simulink model "DC_Motor_BrakeMode"  (R2019b)
settings: Solver=VariableStepAuto  StartTime=0.0  StopTime=10.0  FixedStep=1e-5  RelTol=1e-3
PreLoadFcn:
  | modelDir = fileparts(get_param(bdroot, 'FileName'));
  | addpath(fullfile(modelDir,'../../Parameters'));
  | 
  | Parameters_Model
  | Parameters_Simulation
  | Parameters_Controller
InitFcn:
  | Parameters_Model
  | Parameters_Simulation
  | Parameters_Controller
undefined symbols (not defined in the file): B, dTheta0, I0, J, Ke, Kt, L, R, tau_c, theta0
settings Model: Creator=Thomas  LastModifiedBy=thomas.jespersen
settings DataIOCC: ReturnWorkspaceOutputs=off
settings DebuggingCC: ArithmeticOperatorsInVariantConditions=warning
settings SFSimCC: SimUseLocalCustomCode=off  CustomCodeUndefinedFunction=UseInterfaceOnly
settings RTWCC: RTWUseLocalCustomCode=off

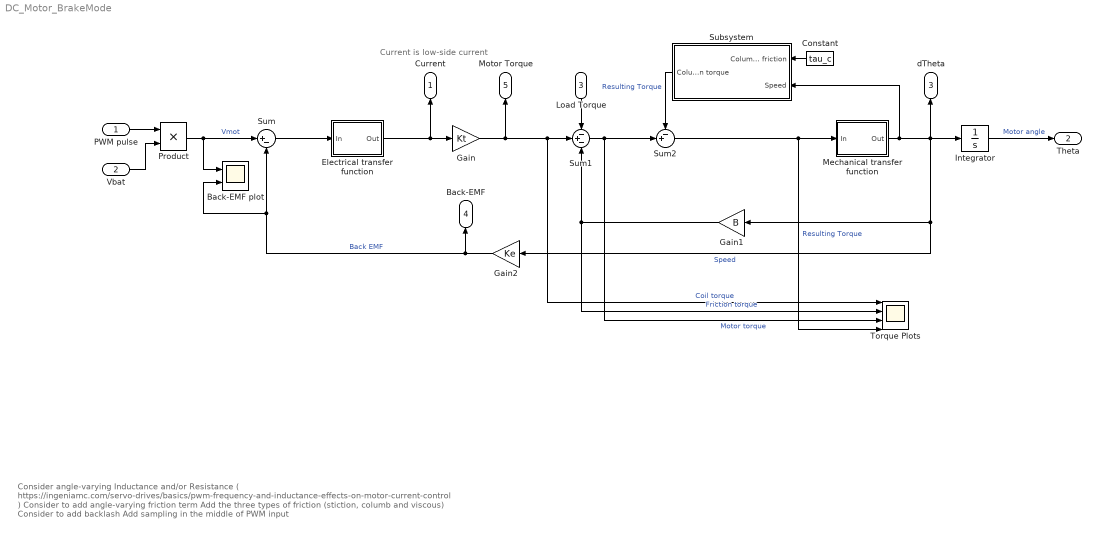
== system DC_Motor_BrakeMode ==
  note: Consider angle-varying Inductance and/or Resistance ( https://ingeniamc.com/servo-drives/basics/pwm-frequency-and-inductance-effects-on-motor-current-control )
      | Consider to add angle-varying friction term
      | Add the three types of friction (stiction, columb and viscous)
      | Consider to add backlash
      | Add sampling in the middle of PWM input
  note: Current is low-side current
  PWM pulse : Inport  OutDataTypeStr=int8
  Vbat : Inport  Port=2  OutDataTypeStr=double
  Load Torque : Inport  Port=3  OutDataTypeStr=double
  Back-EMF plot : Scope  NumInputPorts=2
  Constant : Constant  Value=tau_c
  Electrical transfer function : Subsystem
  Gain : Gain  Gain=Kt
  Gain1 : Gain  Gain=B
  Gain2 : Gain  Gain=Ke
  Integrator : Integrator  InitialCondition=theta0
  Mechanical transfer function : Subsystem
  Product : Product  OutDataTypeStr=double
  Subsystem : Subsystem
  Sum : Sum  Inputs=|+-
  Sum1 : Sum  Inputs=-+-
  Sum2 : Sum  Inputs=-+|
  Torque Plots : Scope  NumInputPorts=4
  Current : Outport  VectorParamsAs1DForOutWhenUnconnected=off
  Theta : Outport  Port=2  VectorParamsAs1DForOutWhenUnconnected=off
  dTheta : Outport  Port=3  VectorParamsAs1DForOutWhenUnconnected=off
  Back-EMF : Outport  Port=4  VectorParamsAs1DForOutWhenUnconnected=off
  Motor Torque : Outport  Port=5  VectorParamsAs1DForOutWhenUnconnected=off
  wires:
  Vbat/1 -> Product/2
  PWM pulse/1 -> Product/1
  Product/1 -> Sum/1, Back-EMF plot/1  "Vmot"
  Electrical transfer function/1(Out) -> Current/1, Gain/1
  Sum/1 -> Electrical transfer function/1(In)
  Gain/1 -> Torque Plots/1, Sum1/2, Motor Torque/1  "Coil torque"
  Load Torque/1 -> Sum1/1
  Sum1/1 -> Torque Plots/3, Sum2/2  "Motor torque"
  Mechanical transfer function/1(Out) -> Subsystem/2(Speed), Gain1/1, Gain2/1, Integrator/1, dTheta/1  "Speed"
  Gain1/1 -> Torque Plots/2, Sum1/3  "Friction torque"
  Integrator/1 -> Theta/1  "Motor angle"
  Gain2/1 -> Sum/2, Back-EMF plot/2, Back-EMF/1  "Back EMF"
  Sum2/1 -> Torque Plots/4, Mechanical transfer function/1(In)  "Resulting Torque"
  Constant/1 -> Subsystem/1(Columb friction)
  Subsystem/1(Columb friction torque) -> Sum2/1  "Resulting Torque"

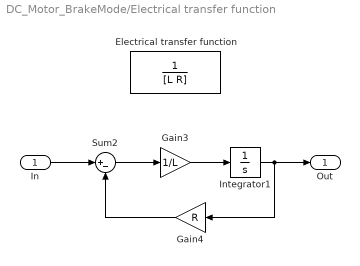
== system DC_Motor_BrakeMode/Electrical transfer function ==
  In : Inport
  Electrical transfer function : TransferFcn  Denominator=[L R]
  Gain3 : Gain  Gain=1/L
  Gain4 : Gain  Gain=R
  Integrator1 : Integrator  InitialCondition=I0
  Sum2 : Sum  Inputs=|+-
  Out : Outport  VectorParamsAs1DForOutWhenUnconnected=off
  wires:
  In/1 -> Sum2/1
  Gain3/1 -> Integrator1/1
  Gain4/1 -> Sum2/2
  Sum2/1 -> Gain3/1
  Integrator1/1 -> Out/1, Gain4/1

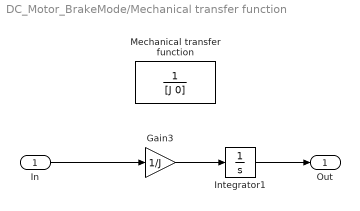
== system DC_Motor_BrakeMode/Mechanical transfer function ==
  In : Inport
  Gain3 : Gain  Gain=1/J
  Integrator1 : Integrator  InitialCondition=dTheta0
  Mechanical transfer function : TransferFcn  Denominator=[J 0]
  Out : Outport  VectorParamsAs1DForOutWhenUnconnected=off
  wires:
  Gain3/1 -> Integrator1/1
  In/1 -> Gain3/1
  Integrator1/1 -> Out/1

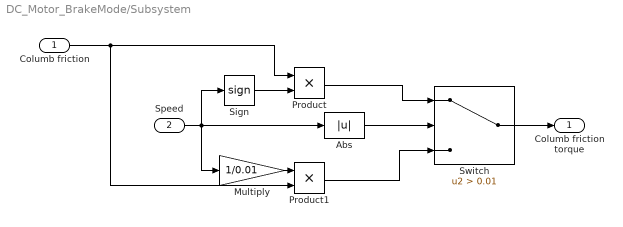
== system DC_Motor_BrakeMode/Subsystem ==
  Columb friction : Inport
  Speed : Inport  Port=2  OutDataTypeStr=double
  Abs : Abs
  Multiply : Gain  Gain=1/0.01
  Product : Product
  Product1 : Product
  Sign : Signum
  Switch : Switch  Criteria=u2 > Threshold  Threshold=0.01
  Columb friction torque : Outport  VectorParamsAs1DForOutWhenUnconnected=off
  wires:
  Abs/1 -> Switch/2
  Speed/1 -> Multiply/1, Sign/1, Abs/1
  Sign/1 -> Product/2
  Product/1 -> Switch/1
  Switch/1 -> Columb friction torque/1
  Multiply/1 -> Product1/1
  Product1/1 -> Switch/3
  Columb friction/1 -> Product1/2, Product/1
